simulink model "DE_epsIn_task_2"  (R2018a)
settings: Solver=ode15s  StartTime=0.0  StopTime=2.5  MaxStep=0.01  RelTol=1e-6  EnableMultiTasking=on
InitFcn:
  | Parameter;
values from neighbouring files (symbols this model uses):
  params = struct    [Parameter.m]
  params_voltage = 0    [task_2_0V.m]    (also in task_2_2000V.m = 2000)
libraries: simulink x1
settings Model: Creator=Johannes  LastModifiedBy=tim
settings DataIOCC: LimitDataPoints=on  SaveFormat=Array  SignalLoggingSaveFormat=ModelDataLogs
settings OptimizationCC: LifeSpan=inf
settings DebuggingCC: UnderspecifiedInitializationDetection=Classic  MergeDetectMultiDrivingBlocksExec=none  SolverPrmCheckMsg=warning  MultiTaskDSMMsg=warning  MultiTaskCondExecSysMsg=none  SFUnexpectedBacktrackingDiag=warning  SFNoUnconditionalDefaultTransitionDiag=warning  SFExecutionAtInitializationDiag=none
settings HardwareCC: ProdBitPerPointer=32  ProdBitPerSizeT=32  ProdBitPerPtrDiffT=32  ProdLargestAtomicFloat=None  ProdIntDivRoundTo=Undefined  ProdEndianess=Unspecified  ProdWordSize=32  ProdHWDeviceType=32-bit Generic
settings ModelReferenceCC: PropagateSignalLabelsOutOfModel=off
settings CodeAppCC: StateflowObjectComments=on
settings GRTTargetCC: TargetLangStandard=C89/C90 (ANSI)  GeneratePreprocessorConditionals=Disable all
settings ConfigComp: CovMetricSettings=dw  CovHtmlReporting=on  CovSaveCumulativeToWorkspaceVar=on  CovSaveSingleToWorkspaceVar=on  CovExternalEMLEnable=off

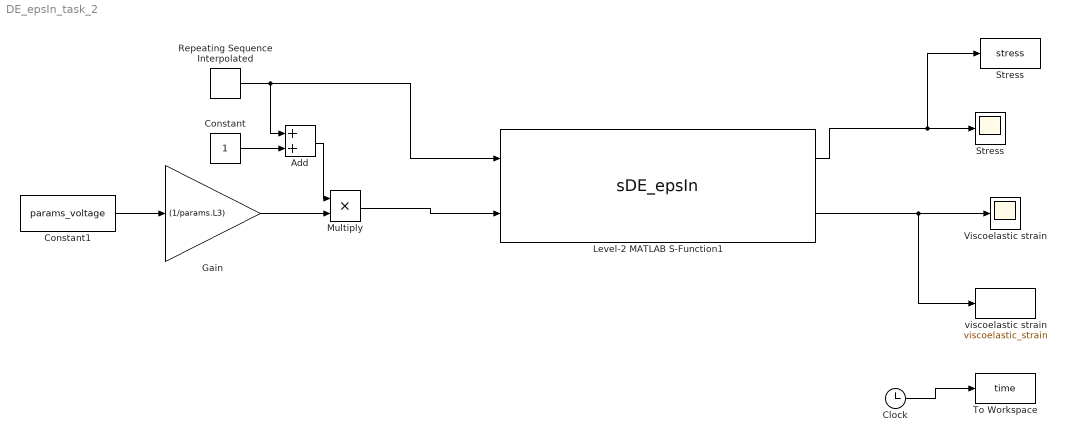
== system DE_epsIn_task_2 ==
  Add : Sum
  Clock : Clock
  Constant : Constant
  Constant1 : Constant  Value=params_voltage
  Gain : Gain  Gain=(1/params.L3)
  Level-2 MATLAB S-Function1 : M-S-Function  FunctionName=sDE_epsIn  Parameters=params, initConds
      mask Display:
      | color('black');
      | patch(4*[-1 1 1 -1],1.75*[-1 -1 1 1],[1 1 1]);
      | patch(2*[-1 1 1 -1],1.2*[-1 -1 1 1],[0 0 0]);
      | patch(1.95*[-1 1 1 -1],0.8*[-1 -1 1 1],[1 1 1]);
      | disp('DE');
      | 
      | color('blue');
      | port_label('input', 1, '\epsilon [-]','texmode','on');
      | port_label('input', 2, 'E [V/m]','texmode','on');
      | 
      | color('red');
      | port_label('output', 1, '\sigma [Pa]','texmode','on');
      | port_label('output', 2, 'x_v [-]','texmode','on');
  Multiply : Product
  Repeating Sequence Interpolated : simulink/Sources/Repeating Sequence Interpolated  OutValues=strain  TimeValues=time  LookUpMeth=Interpolation-Use End Values  tsamp=0.001  OutMin=[]  OutMax=[]  OutDataTypeStr=double  OutputDataTypeScalingMode=double  OutDataType=fixdt(0,8)  OutScaling=2^-10
  Stress : Scope
  "Stress " : ToWorkspace  VariableName=stress  SampleTime=-1
  To Workspace : ToWorkspace  VariableName=time  SampleTime=-1
  Viscoelastic strain : Scope
  "viscoelastic strain " : ToWorkspace  VariableName=viscoelastic_strain  SampleTime=-1
  wires:
  Repeating Sequence Interpolated/1 -> Add/1, Level-2 MATLAB S-Function1/1
  Level-2 MATLAB S-Function1/1 -> "Stress "/1, Stress/1
  Level-2 MATLAB S-Function1/2 -> "viscoelastic strain "/1, Viscoelastic strain/1
  Constant1/1 -> Gain/1
  Clock/1 -> To Workspace/1
  Gain/1 -> Multiply/2
  Multiply/1 -> Level-2 MATLAB S-Function1/2
  Constant/1 -> Add/2
  Add/1 -> Multiply/1
